simulink model "Q6"  (R2022a)
settings: Solver=VariableStepAuto  StartTime=0.0  StopTime=0.003  RelTol=1e-3
undefined symbols (not defined in the file): A, B, C, K, L1
settings Model: Creator=fatae  LastModifiedBy=fatae

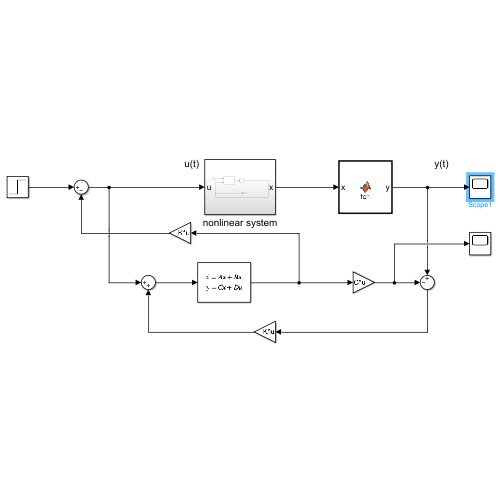
[thumbnail: Simulink's stored preview of the top-level diagram]
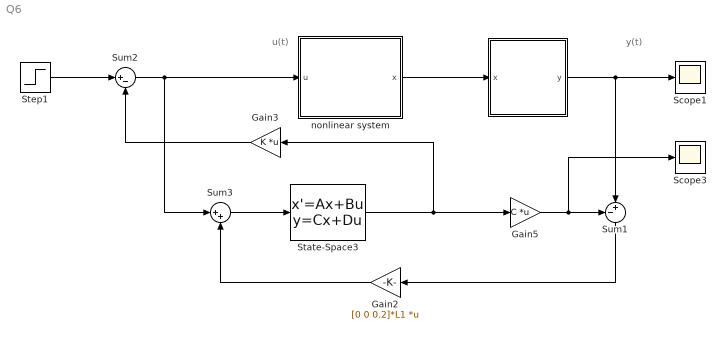
== system Q6 ==
  note: y(t)
  note: u(t)
  "  " : MATLAB Function  TreatAsAtomicUnit=on
  Gain2 : Gain  Gain=[0 0 0.2]*L1  Multiplication=Matrix(K*u)
  Gain3 : Gain  Gain=K  Multiplication=Matrix(K*u)
  Gain5 : Gain  Gain=C  Multiplication=Matrix(K*u)
  Scope1 : Scope
  Scope3 : Scope
  State-Space3 : StateSpace  A=A  B=B  C=[1 0 0; 0 1 0;0 0 1]  D=[0;0;0]  InitialCondition=0
  Step1 : Step  Time=0  SampleTime=0
  Sum1 : Sum  Inputs=-+|
  Sum2 : Sum  Inputs=|+-
  Sum3 : Sum  Inputs=|++
  nonlinear system : Subsystem
  wires:
  Sum1/1 -> Gain2/1
  Step1/1 -> Sum2/1
  Gain2/1 -> Sum3/2
  Sum3/1 -> State-Space3/1
  Gain3/1 -> Sum2/2
  State-Space3/1 -> Gain3/1, Gain5/1
  Gain5/1 -> Scope3/1, Sum1/1
  "  "/1(y) -> Sum1/2, Scope1/1
  Sum2/1 -> Sum3/1, nonlinear system/1(u)
  nonlinear system/1(x) -> "  "/1(x)

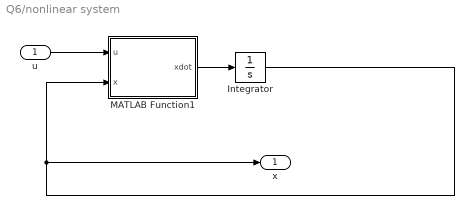
== system Q6/nonlinear system ==
  u : Inport
  Integrator : Integrator  InitialCondition=[0.01;0;0.3]
  MATLAB Function1 : MATLAB Function  TreatAsAtomicUnit=on
  x : Outport  VectorParamsAs1DForOutWhenUnconnected=off
  wires:
  u/1 -> MATLAB Function1/1(u)
  MATLAB Function1/1(xdot) -> Integrator/1
  Integrator/1 -> x/1, MATLAB Function1/2(x)

== matlab function Q6/nonlinear system/MATLAB Function1 ==
  settings: updateMethod=DISCRETE  sampleTime=1e-6
  data: u input; x input; xdot output
function xdot = EQofMotion(u,x)
    if isempty(x)
        x=[0.01;0;0];
    end
    if isempty(u)
        u=0;
    end
    R = 50; 
    L = 0.2; 
    g = 9.8; 
    M = 0.4+0.079; 
    c = 0.3; 
    fv = 0.04; 

    xdot=[0;0;0];
    xdot(1)=x(2);   
    xdot(2)= g-c*(x(3)^2)/(M*(0.1-x(1)))-fv*x(2)/M; 
    xdot(3)=1/L*(-(R)*x(3)+u);
end

== matlab function Q6/   ==
  settings: updateMethod=DISCRETE  sampleTime=1e-6
  data: x input; y output
function y = fcn(x)
y=0;
C=[1 0 0];
y=C*x;
